simulink model "bike_model_old"  (R2018b)
settings: Solver=VariableStepAuto  StartTime=0.0  StopTime=sim_time  FixedStep=Ts_IMU  MaxStep=Ts  RelTol=1e-3
values from neighbouring files (symbols this model uses):
  a_compFilter = b_compFilter - 0.77    (= 0.325)    [configuration.m]    (also in configuration_pidTuning.m)
  A_kalman = [1 0 Ts 0; 0 1 0 Ts; 0 0 1 0; 0 0 0 1]    [configuration.m]    (also in configuration_pidTuning.m)
  b_compFilter = 1.095    [configuration.m]    (also in configuration_pidTuning.m)
  B_kalman = [0 0 0 0; 0 0 0 0; 0 0 0 0; 0 0 0 0]    [configuration.m]    (also in configuration_pidTuning.m)
  b_real = 1.095    [configuration.m]    (also in configuration_pidTuning.m)
  C_kalman = [1 0 0 0; 0 1 0 0; 0 0 1 0; 0 0 0 1]    [configuration.m]    (also in configuration_pidTuning.m)
  complementary = 0.985    [configuration.m]    (also in configuration_pidTuning.m)
  D_kalman = [0 0 0 0; 0 0 0 0; 0 0 0 0; 0 0 0 0]    [configuration.m]    (also in configuration_pidTuning.m)
  Dead_Band = [0.055, -0.055, 0.005]    [configuration.m]    (also in configuration_pidTuning.m)
  delay = 0.045    [configuration.m]    (also in configuration_pidTuning.m)
  direct_control = 1    [configuration.m]    (also in configuration_pidTuning.m)
  filter_model = 1    [configuration.m]    (also in configuration_pidTuning.m)
  forward_motor_dynamics = 0    [configuration.m]    (also in configuration_pidTuning.m)
  forward_speed_offset = 0    [configuration.m]
  g = 9.81    [configuration.m]    (also in configuration_pidTuning.m)
  I_direct = 0.000227125326188444    (= 0.000227125326188)    [configuration.m]    (also in configuration_pidTuning.m)
  I_lat = 0.000115580509653549    (= 0.000115580509654)    [configuration.m]    (also in configuration_pidTuning.m)
  I_steer = 0.4510120195392    (= 0.451012019539)    [configuration.m]    (also in configuration_pidTuning.m)
  IMU_height_model = 0.45    [configuration.m]    (also in configuration_pidTuning.m)
  IMU_height_real = 0.45    [configuration.m]    (also in configuration_pidTuning.m)
  initial_states = [deg2rad(-2) deg2rad(0) deg2rad(0)]    [configuration.m]    (also in configuration_pidTuning.m)
  input_velocity = 4    [configuration.m]    (also in configuration_pidTuning.m = 3)
  K_dir = [0.2 0 0]    [configuration.m]
  K_pos = [0.02 0 0]    [configuration.m]
  lambda_compFilter = deg2rad(70)    [configuration.m]    (also in configuration_pidTuning.m)
  lambda_real = deg2rad(70)    [configuration.m]    (also in configuration_pidTuning.m)
  lat_control = 0    [configuration.m]    (also in configuration_pidTuning.m = 1)
  look_ahead = 0    [configuration.m]    (also in configuration_pidTuning.m)
  lqr_gains = zeros(length(velocity_lqr),1+size(A_bike,1))    [lqr_design.m]
  max_handlebar = 40*(pi/180)    (= 0.698131700798)    [configuration.m]    (also in configuration_pidTuning.m)
  max_roll = pi/2    (= 1.57079632679)    [configuration.m]    (also in configuration_pidTuning.m)
  max_steering_motor_acc = inf    [configuration.m]    (also in configuration_pidTuning.m)
  max_steering_motor_speed = 0.9    [configuration.m]    (also in configuration_pidTuning.m = 7.5)
  min_handlebar = -max_handlebar    (= -0.698131700798)    [configuration.m]    (also in configuration_pidTuning.m)
  min_roll = - max_roll    (= -1.57079632679)    [configuration.m]    (also in configuration_pidTuning.m)
  min_steering_motor_acc = -inf    [configuration.m]    (also in configuration_pidTuning.m)
  min_steering_motor_speed = -0.9    [configuration.m]    (also in configuration_pidTuning.m = -7.5)
  noise = 0    [configuration.m]    (also in configuration_pidTuning.m)
  noise_acc = 2.4869e-05    [configuration.m]    (also in configuration_pidTuning.m)
  noise_encoder = 1e-7    (= 1e-07)    [configuration.m]    (also in configuration_pidTuning.m)
  noise_gyro = 0.005    [configuration.m]    (also in configuration_pidTuning.m = 0.0022)
  noise_hall = 0.0031    [configuration.m]    (also in configuration_pidTuning.m)
  noise_pos_meas = 0    [configuration.m]    (also in configuration_pidTuning.m = 0.51)
  offset_acc = 0.0*g    (= 0)    [configuration.m]
  offset_encoder = deg2rad(1)    [configuration.m]
  offset_gyro = deg2rad(0)    [configuration.m]
  offset_hall = 0.0    (= 0)    [configuration.m]
  offset_pos_x = 0    [configuration.m]
  offset_pos_y = 0    [configuration.m]
  P_direct = 0.0712859744206787    (= 0.0712859744207)    [configuration.m]    (also in configuration_pidTuning.m)
  P_lat = 0.0465435246389258    (= 0.0465435246389)    [configuration.m]    (also in configuration_pidTuning.m)
  P_steer = 0.219020351848633    (= 0.219020351849)    [configuration.m]    (also in configuration_pidTuning.m)
  parameters_compFilter = [g h_compFilter b_compFilter a_compFilter lambda_compFilter c_compFilter]    [configuration.m]    (also in configuration_pidTuning.m)
  parameters_f_b_real = [m_frame_real m_box_real h_frame_real h_box_real a_frame_real a_box_real c_frame_real c_box_real b_frame_real b_box_real l_frame_real l_box_real]    [configuration.m]    (also in configuration_pidTuning.m)
  parameters_real = [g h_real b_real a_real lambda_real c_real]    [configuration.m]    (also in configuration_pidTuning.m)
  path_tracking = 0    [configuration.m]    (also in configuration_pidTuning.m = 1)
  plant_model = 2    [configuration.m]    (also in configuration_pidTuning.m = 1)
  R_kalman = [noise_pos_meas 0 0 0; 0 noise_pos_meas 0 0; 0 0 noise_hall 0; 0 0 0 noise_hall]    [configuration.m]    (also in configuration_pidTuning.m)
  roll_rate_coef = 0.9    [configuration.m]    (also in configuration_pidTuning.m)
  sensor_offset = 0    [configuration.m]
  steer_control = 0    [configuration.m]    (also in configuration_pidTuning.m = 1)
  steering_angle_correction = deg2rad(0)    [configuration.m]
  steering_motor_limitations = 0    [configuration.m]    (also in configuration_pidTuning.m = 1)
  sys_con = ss(A_lqr,B_lqr,C_lqr,D_lqr)    [lqr_design.m]
  sys_dis = c2d(sys_con,Ts)    [lqr_design.m]
  time_offset_acc = 7    [configuration.m]
  time_offset_encoder = 10    [configuration.m]
  time_offset_gyro = 7    [configuration.m]
  time_offset_hall = 7    [configuration.m]
  time_offset_pos_x = 7    [configuration.m]
  time_offset_pos_y = 7    [configuration.m]
  Ts = 0.01    [configuration.m]    (also in configuration_pidTuning.m = 0.04)
  Ts_IMU = 0.01    [configuration.m]    (also in configuration_pidTuning.m = 0.04)
  uneven_mass = 0    [configuration.m]
  velocity_lqr = [input_velocity - 0.1 , input_velocity , input_velocity + 0.1]    [lqr_design.m]
undefined symbols (not defined in the file or in its folder): A, B, cumulative_dist_along_path, curvature, DiscIntNeverNeededParam, Discrete, initial_x, initial_y, path_x, path_y, Time
libraries: simulink x23, simulink_extras x4, dspsigops x2, ctrlSharedLib x1
(part 1 of 3)
settings Model: Creator=Boaz Ash  LastModifiedBy=maximef
settings DebuggingCC: UnconnectedInputMsg=none  UnconnectedOutputMsg=none  UnconnectedLineMsg=none  LibraryContextMissingDiagnostic=none
settings SFSimCC: SimUseLocalCustomCode=off
settings RTWCC: RTWUseLocalCustomCode=off

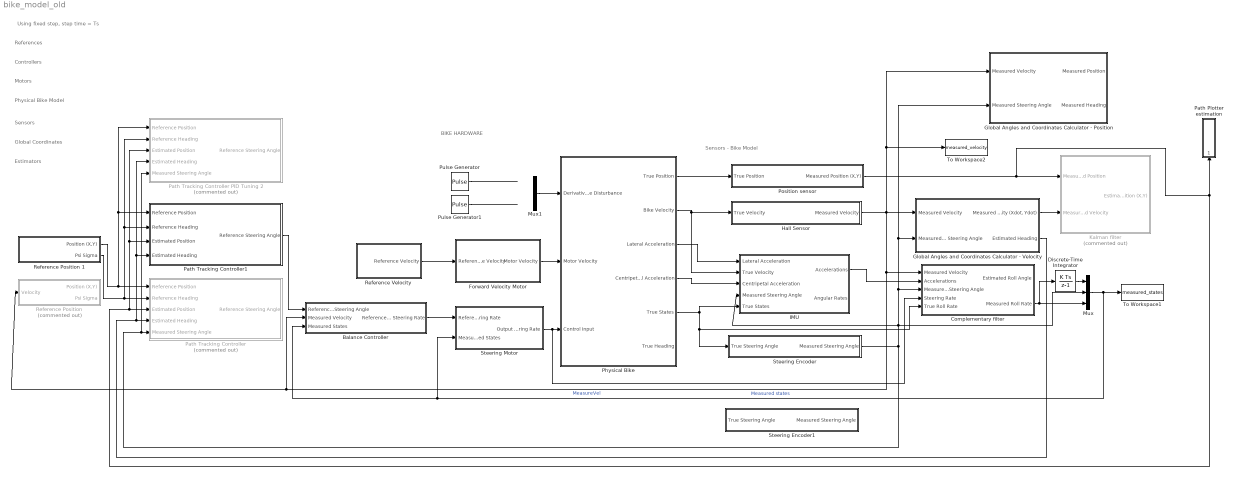
== system bike_model_old ==
  note: Using fixed step, step time = Ts
  note: BIKE HARDWARE
  note: References
  note: Physical Bike
      | Model
  note: Sensors - Bike Model
  note: Motors
  note: Sensors
  note: Global Coordinates
  note: Controllers
  note: Estimators
  Balance Controller : Subsystem  TreatAsAtomicUnit=on  SystemSampleTime=Ts
  Complementary filter : Subsystem  SystemSampleTime=Ts_IMU
  Discrete-Time Integrator : DiscreteIntegrator  SampleTime=Ts  ICPrevOutput=DiscIntNeverNeededParam  ICPrevScaledInput=DiscIntNeverNeededParam
  Forward Velocity Motor : Subsystem
  Global Angles and Coordinates Calculator - Position : Subsystem  SystemSampleTime=Ts
  Global Angles and Coordinates Calculator - Velocity : Subsystem  SystemSampleTime=Ts
  Hall Sensor : Subsystem  TreatAsAtomicUnit=on  SystemSampleTime=Ts
  IMU : Subsystem  TreatAsAtomicUnit=on
  "Kalman filter " : Subsystem  Commented=on  SystemSampleTime=Ts
  Mux : Mux  Inputs=3
  Mux1 : Mux  Inputs=3
  Path Plotter estimation : Subsystem  SystemSampleTime=Ts
  Path Tracking Controller : Subsystem  Commented=on
  Path Tracking Controller PID Tuning 2 : Subsystem  Commented=on
  Path Tracking Controller1 : Subsystem
  Physical Bike : Subsystem
  Position sensor : Subsystem  TreatAsAtomicUnit=on  SystemSampleTime=Ts
  Pulse Generator : DiscretePulseGenerator  PulseType=Time based  Amplitude=pi/36  Period=100  PhaseDelay=1
  Pulse Generator1 : DiscretePulseGenerator  PulseType=Time based  Amplitude=-deg2rad(30)  Period=10  PulseWidth=10  PhaseDelay=1
  "Reference Position " : Subsystem  Commented=on
  Reference Position 1 : Subsystem
  "Reference Velocity " : Subsystem
  Steering Encoder : Subsystem  TreatAsAtomicUnit=on  SystemSampleTime=Ts
  Steering Encoder1 : Subsystem  TreatAsAtomicUnit=on  SystemSampleTime=Ts
  Steering Motor : Subsystem
  To Workspace1 : ToWorkspace  VariableName=measured_states  SaveFormat=Timeseries  SampleTime=-1
  To Workspace2 : ToWorkspace  VariableName=measured_velocity  SaveFormat=Timeseries  SampleTime=-1
  wires:
  Mux1/1 -> Physical Bike/1(Derivative Disturbance)
  "Reference Velocity "/1(Reference Velocity) -> Forward Velocity Motor/1(Reference Velocity)
  Forward Velocity Motor/1(Motor Velocity) -> Physical Bike/2(Motor Velocity)
  Pulse Generator/1 -> ?
  Pulse Generator1/1 -> ?
  Position sensor/1("Measured Position (X,Y) ") -> Path Tracking Controller1/3(Estimated Position), Path Tracking Controller PID Tuning 2/3(Estimated Position), Path Tracking Controller/3(Estimated Position), Path Plotter estimation/1(Position), "Kalman filter "/1("Measured Position ")
  Global Angles and Coordinates Calculator - Velocity/2(Estimated Heading) -> Path Tracking Controller PID Tuning 2/4(Estimated Heading), Path Tracking Controller1/4(Estimated Heading), Path Tracking Controller/4(Estimated Heading)
  Path Tracking Controller1/1(Reference Steering Angle) -> Balance Controller/1(Reference Steering Angle)
  Balance Controller/1(Reference Steering Rate) -> Steering Motor/1(Reference Steering Rate)
  Physical Bike/3(Lateral Acceleration) -> IMU/1(Lateral Acceleration)
  Physical Bike/4(Centripetal Acceleration) -> IMU/3(Centripetal Acceleration)
  Mux/1 -> To Workspace1/1, Steering Motor/2(Measured States), Balance Controller/3(Measured States)  "Measured states"
  Steering Encoder/1(Measured Steering Angle) -> Global Angles and Coordinates Calculator - Position/2(Measured Steering Angle), Global Angles and Coordinates Calculator - Velocity/2("Measured Steering Angle "), Complementary filter/3(Measured Steering Angle), Mux/2, IMU/4(Measured Steering Angle), Path Tracking Controller PID Tuning 2/5(Measured Steering Angle), Path Tracking Controller/5(Measured Steering Angle)
  IMU/1(Accelerations) -> Complementary filter/2(Accelerations)
  Global Angles and Coordinates Calculator - Velocity/1("Measured Velocity (Xdot, Ydot)") -> "Kalman filter "/2(Measured Velocity)
  Hall Sensor/1(Measured Velocity) -> Global Angles and Coordinates Calculator - Position/1(Measured Velocity), To Workspace2/1, Complementary filter/1(Measured Velocity), Balance Controller/2(Measured Velocity), "Reference Position "/1(Velocity), Global Angles and Coordinates Calculator - Velocity/1(Measured Velocity)  "MeasureVel"
  Reference Position 1/2(Psi Sigma) -> Path Tracking Controller1/2(Reference Heading), Path Tracking Controller PID Tuning 2/2(Reference Heading), Path Tracking Controller/2(Reference Heading)
  Reference Position 1/1(Position (X,Y)) -> Path Tracking Controller PID Tuning 2/1(Reference Position), Path Tracking Controller1/1(Reference Position), Path Tracking Controller/1(Reference Position)
  Physical Bike/2(Bike Velocity) -> IMU/2(True Velocity), Hall Sensor/1(True Velocity)
  Physical Bike/1(True Position) -> Position sensor/1(True Position)
  Steering Motor/1(Output Steering Rate) -> Complementary filter/4(Steering Rate), Physical Bike/3(Control Input)
  Physical Bike/5(True States) -> Complementary filter/5(True Roll Rate), Steering Encoder/1(True Steering Angle), IMU/5(True States)
  Complementary filter/2(Measured Roll Rate) -> Mux/3, Discrete-Time Integrator/1
  Discrete-Time Integrator/1 -> Mux/1

== system bike_model_old/Balance Controller ==
  Reference Steering Angle : Inport
  Measured Velocity : Inport  Port=2
  Measured States : Inport  Port=3
  LQR Controller : Subsystem  TreatAsAtomicUnit=on  SystemSampleTime=Ts
  Reference States : Subsystem  SystemSampleTime=Ts
  Sum : Sum  Inputs=|+-
  To Workspace : ToWorkspace  VariableName=states_measured  SaveFormat=Timeseries  SampleTime=-1
  Reference Steering Rate : Outport
  wires:
  Reference States/1(Reference States) -> Sum/1
  Sum/1 -> LQR Controller/2(State Error)
  LQR Controller/1(Calculated Input) -> Reference Steering Rate/1
  Measured Velocity/1 -> Reference States/1(Velocity), LQR Controller/1(Velocity)
  Measured States/1 -> To Workspace/1, Sum/2
  Reference Steering Angle/1 -> Reference States/2(Delta Ref)

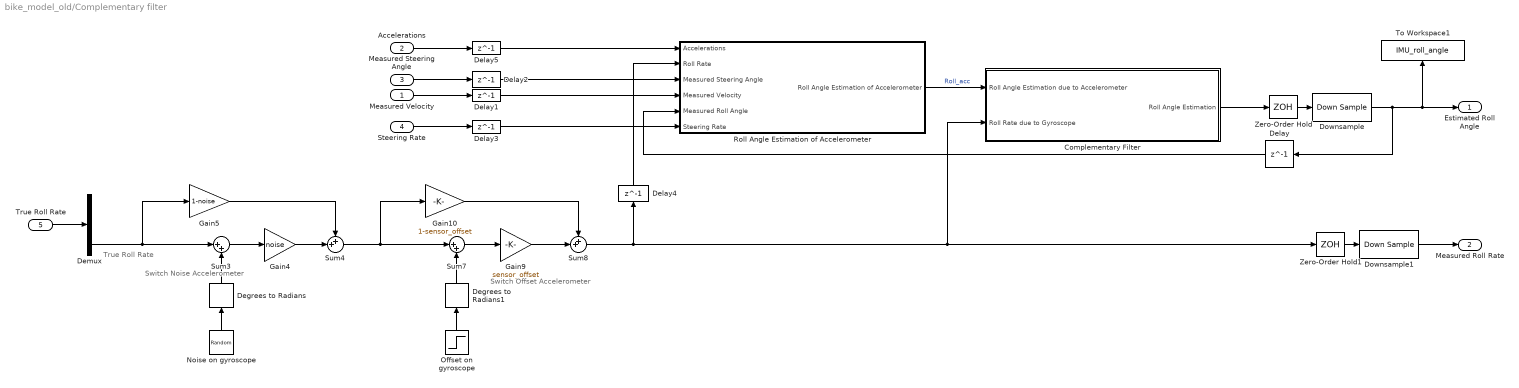
== system bike_model_old/Complementary filter ==
  note: Switch Noise
      | Accelerometer
  note: True Roll
      | Rate
  note: Switch Offset
      | Accelerometer
  Measured Velocity : Inport
  Accelerations : Inport  Port=2
  Measured Steering Angle : Inport  Port=3
  Steering Rate : Inport  Port=4
  True Roll Rate : Inport  Port=5
  Complementary Filter : Subsystem  TreatAsAtomicUnit=on  SystemSampleTime=Ts_IMU
  Degrees to Radians : simulink_extras/Transformations/Degrees to Radians
  Degrees to Radians1 : simulink_extras/Transformations/Degrees to Radians
  Delay{,1..2,4..5} (5 alike) : Delay  DelayLength=1
  Delay3 : Delay  DelayLength=1  SampleTime=Ts_IMU
  Demux : Demux  Outputs=3
  Downsample : DownSample  N=Ts/Ts_IMU  RateOptions=Allow multirate processing
  Downsample1 : DownSample  N=Ts/Ts_IMU  RateOptions=Allow multirate processing
  Gain10 : Gain  Gain=1-sensor_offset
  Gain4 : Gain  Gain=noise
  Gain5 : Gain  Gain=1-noise
  Gain9 : Gain  Gain=sensor_offset
  Noise on gyroscope : RandomNumber  Variance=noise_gyro  SampleTime=Ts
  Offset on gyroscope : Step  Time=time_offset_gyro  After=offset_gyro  SampleTime=Ts
  Roll Angle Estimation of Accelerometer : Subsystem
  Sum3 : Sum  Inputs=|++
  Sum4 : Sum  Inputs=++|
  Sum7 : Sum  Inputs=|++
  Sum8 : Sum  Inputs=++|
  To Workspace1 : ToWorkspace  VariableName=IMU_roll_angle  SaveFormat=Structure  SampleTime=-1
  Zero-Order Hold : ZeroOrderHold  SampleTime=Ts_IMU
  Zero-Order Hold1 : ZeroOrderHold  SampleTime=Ts_IMU
  Estimated Roll Angle : Outport
  Measured Roll Rate : Outport  Port=2
  wires:
  Roll Angle Estimation of Accelerometer/1(Roll Angle Estimation of Accelerometer) -> Complementary Filter/1(Roll Angle Estimation due to Accelerometer)  "Roll_acc"
  Sum8/1 -> Zero-Order Hold1/1, Complementary Filter/2(Roll Rate due to Gyroscope), Delay4/1
  Zero-Order Hold/1 -> Downsample/1
  Zero-Order Hold1/1 -> Downsample1/1
  Accelerations/1 -> Delay5/1
  Measured Steering Angle/1 -> Delay2/1
  Measured Velocity/1 -> Delay1/1
  Delay/1 -> Roll Angle Estimation of Accelerometer/5(Measured Roll Angle)
  Delay1/1 -> Roll Angle Estimation of Accelerometer/4(Measured Velocity)
  Delay2/1 -> Roll Angle Estimation of Accelerometer/3(Measured Steering Angle)
  Steering Rate/1 -> Delay3/1
  Delay3/1 -> Roll Angle Estimation of Accelerometer/6(Steering Rate)
  Delay4/1 -> Roll Angle Estimation of Accelerometer/2(Roll Rate)
  Delay5/1 -> Roll Angle Estimation of Accelerometer/1(Accelerations)
  Complementary Filter/1(Roll Angle Estimation) -> Zero-Order Hold/1
  Downsample1/1 -> Measured Roll Rate/1
  Downsample/1 -> Estimated Roll Angle/1, To Workspace1/1, Delay/1
  Demux/3 -> Sum3/1, Gain5/1
  Sum3/1 -> Gain4/1
  Noise on gyroscope/1 -> Degrees to Radians/1
  Gain4/1 -> Sum4/2
  Gain5/1 -> Sum4/1
  Degrees to Radians/1 -> Sum3/2
  True Roll Rate/1 -> Demux/1
  Gain9/1 -> Sum8/2
  Sum7/1 -> Gain9/1
  Sum4/1 -> Gain10/1, Sum7/1
  Degrees to Radians1/1 -> Sum7/2
  Offset on gyroscope/1 -> Degrees to Radians1/1
  Gain10/1 -> Sum8/1

== system bike_model_old/Forward Velocity Motor ==
  note: Add limit for acceleration/deceleration
      | Add min speed of 1.69 m/s (3600 rpm motor speed) limitation
      | Add min speed of 8.20 m/s (18000 rpm motor speed) limitation
      | Add deadband and delay
  Reference Velocity : Inport
  Band-Limited White Noise : simulink/Sources/Band-Limited White Noise  Cov=[0.001]  Ts=Ts  seed=[23341]
  Constant : Constant  Value=forward_motor_dynamics
  Rate Limiter : RateLimiter  RisingSlewLimit=inf  FallingSlewLimit=-inf  SampleTimeMode=inherited
  Saturation : Saturate  UpperLimit=inf  LowerLimit=0
  Sum : Sum  Inputs=|++
  Switch : Switch  Criteria=u2 > Threshold
  Transfer Fcn : TransferFcn  Numerator=[-0.2156 0.556]  Denominator=[1 1.675 0.5558]
  Motor Velocity : Outport
  wires:
  Reference Velocity/1 -> Transfer Fcn/1, Switch/3
  Transfer Fcn/1 -> Rate Limiter/1
  Switch/1 -> Sum/1
  Constant/1 -> Switch/2
  Saturation/1 -> Switch/1
  Rate Limiter/1 -> Saturation/1
  Sum/1 -> Motor Velocity/1

== system bike_model_old/Global Angles and Coordinates Calculator - Position ==
  note: True Steering
      | Angle
  Measured Velocity : Inport
  Measured Steering Angle : Inport  Port=2
  Gain1 : Gain  Gain=sin(lambda_compFilter)
  Measured Bike Angles to Global Angles : Subsystem
  Measured Global Angles to Global Coordinates : Subsystem
  Sum : Sum  Inputs=++|
  Measured Position : Outport
  Measured Heading : Outport  Port=2
  wires:
  Measured Bike Angles to Global Angles/1(Psi) -> Sum/2, Measured Global Angles to Global Coordinates/2(Psi)
  Gain1/1 -> Measured Bike Angles to Global Angles/2(Measured Steering Angle)
  Sum/1 -> Measured Heading/1
  Measured Bike Angles to Global Angles/2(Beta) -> Sum/1, Measured Global Angles to Global Coordinates/3(Beta)
  Measured Global Angles to Global Coordinates/1("Position (X, Y)") -> Measured Position/1
  Measured Velocity/1 -> Measured Global Angles to Global Coordinates/1(Velocity), Measured Bike Angles to Global Angles/1(Velocity)
  Measured Steering Angle/1 -> Gain1/1

== system bike_model_old/Global Angles and Coordinates Calculator - Velocity ==
  Measured Velocity : Inport
  "Measured Steering Angle " : Inport  Port=2
  Gain1 : Gain  Gain=sin(lambda_compFilter)
  Measured Bike Angles to Global Angles : Subsystem
  Measured Global Angles to Global Coordinates : Subsystem
  Sum : Sum  Inputs=++|
  "Measured Velocity (Xdot, Ydot)" : Outport
  Estimated Heading : Outport  Port=2
  wires:
  "Measured Steering Angle "/1 -> Gain1/1
  Measured Bike Angles to Global Angles/1(Psi) -> Sum/2, Measured Global Angles to Global Coordinates/2(Psi)
  Gain1/1 -> Measured Bike Angles to Global Angles/2(Measured Steering Angle)
  Sum/1 -> Estimated Heading/1
  Measured Bike Angles to Global Angles/2(Beta) -> Measured Global Angles to Global Coordinates/3(Beta), Sum/1
  Measured Velocity/1 -> Measured Bike Angles to Global Angles/1(Velocity), Measured Global Angles to Global Coordinates/1(Velocity)
  Measured Global Angles to Global Coordinates/1("Velocity (Xdot, Ydot)") -> "Measured Velocity (Xdot, Ydot)"/1

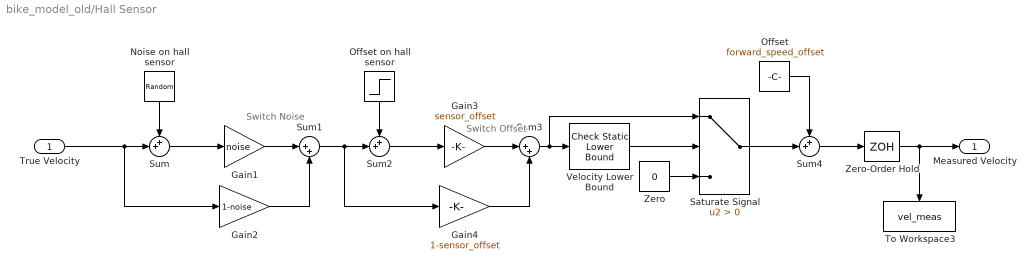
== system bike_model_old/Hall Sensor ==
  note: Switch Noise
  note: Switch Offset
  True Velocity : Inport
  Gain1 : Gain  Gain=noise
  Gain2 : Gain  Gain=1-noise
  Gain3 : Gain  Gain=sensor_offset
  Gain4 : Gain  Gain=1-sensor_offset
  Noise on hall sensor : RandomNumber  Variance=noise_hall  SampleTime=Ts
  Offset : Constant  Value=forward_speed_offset
  Offset on hall sensor : Step  Time=time_offset_hall  After=offset_hall  SampleTime=Ts
  Saturate Signal : Switch  Criteria=u2 > Threshold
  Sum : Sum  Inputs=++|
  Sum1 : Sum  Inputs=|++
  Sum2 : Sum  Inputs=++|
  Sum3 : Sum  Inputs=|++
  Sum4 : Sum  Inputs=++|
  To Workspace3 : ToWorkspace  VariableName=vel_meas  SaveFormat=Timeseries  SampleTime=-1
  Velocity Lower Bound : simulink/Model Verification/Check Static  Lower Bound  Description=0.6 <= u  min=0.6  min_included=on  enabled=on  stopWhenAssertionFail=off  export=on  icon=graphic
      settings: SourceProductName=Simulink
  Zero : Constant  Value=0
  Zero-Order Hold : ZeroOrderHold  SampleTime=Ts
  Measured Velocity : Outport
  wires:
  Sum3/1 -> Saturate Signal/1, Velocity Lower Bound/1
  Noise on hall sensor/1 -> Sum/1
  Zero/1 -> Saturate Signal/3
  Velocity Lower Bound/1 -> Saturate Signal/2
  True Velocity/1 -> Gain2/1, Sum/2
  Gain1/1 -> Sum1/1
  Gain2/1 -> Sum1/2
  Sum/1 -> Gain1/1
  Sum1/1 -> Gain4/1, Sum2/2
  Sum2/1 -> Gain3/1
  Gain4/1 -> Sum3/2
  Gain3/1 -> Sum3/1
  Offset on hall sensor/1 -> Sum2/1
  Sum4/1 -> Zero-Order Hold/1
  Offset/1 -> Sum4/1
  Saturate Signal/1 -> Sum4/2
  Zero-Order Hold/1 -> To Workspace3/1, Measured Velocity/1

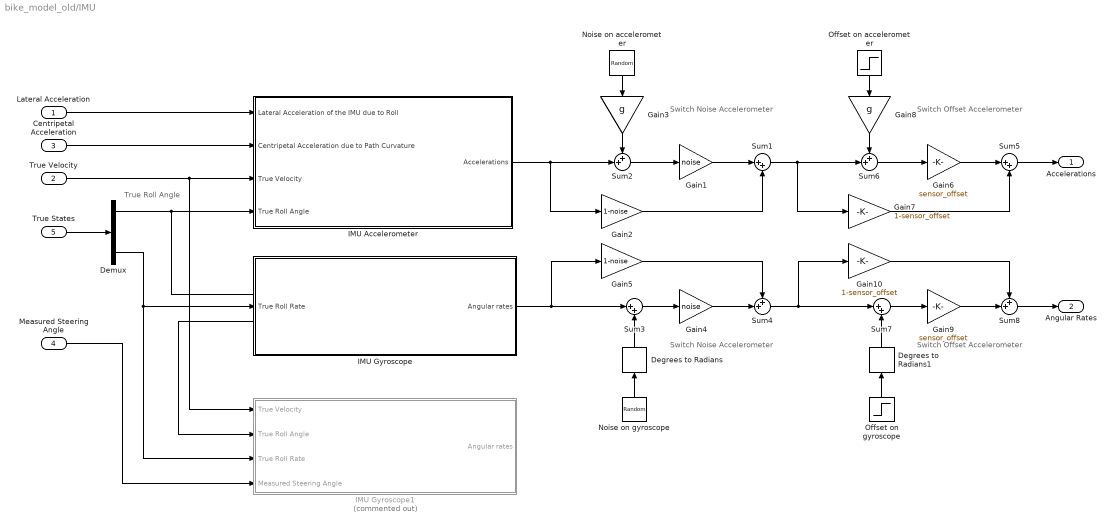
== system bike_model_old/IMU ==
  note: True Roll
      | Angle
  note: Switch Noise
      | Accelerometer
  note: Switch Noise
      | Accelerometer
  note: Switch Offset
      | Accelerometer
  note: Switch Offset
      | Accelerometer
  Lateral Acceleration : Inport
  True Velocity : Inport  Port=2
  Centripetal Acceleration : Inport  Port=3
  Measured Steering Angle : Inport  Port=4
  True States : Inport  Port=5
  Degrees to Radians : simulink_extras/Transformations/Degrees to Radians
  Degrees to Radians1 : simulink_extras/Transformations/Degrees to Radians
  Demux : Demux  Outputs=3
  Gain1 : Gain  Gain=noise
  Gain10 : Gain  Gain=1-sensor_offset
  Gain2 : Gain  Gain=1-noise
  Gain3 : Gain  Gain=g
  Gain4 : Gain  Gain=noise
  Gain5 : Gain  Gain=1-noise
  Gain6 : Gain  Gain=sensor_offset
  Gain7 : Gain  Gain=1-sensor_offset
  Gain8 : Gain  Gain=g
  Gain9 : Gain  Gain=sensor_offset
  IMU Accelerometer : Subsystem
  IMU Gyroscope : Subsystem
  IMU Gyroscope1 : Subsystem  Commented=on
  Noise on accelerometer : RandomNumber  Variance=noise_acc  SampleTime=Ts
  Noise on gyroscope : RandomNumber  Variance=noise_gyro  SampleTime=Ts
  Offset on accelerometer : Step  Time=time_offset_acc  After=offset_acc  SampleTime=Ts
  Offset on gyroscope : Step  Time=time_offset_gyro  After=offset_gyro  SampleTime=Ts
  Sum{1,3,5,7} (4 alike) : Sum  Inputs=|++
  Sum{2,4,6,8} (4 alike) : Sum  Inputs=++|
  Accelerations : Outport
  Angular Rates : Outport  Port=2
  wires:
  Measured Steering Angle/1 -> IMU Gyroscope1/4(Measured Steering Angle)
  True Velocity/1 -> IMU Gyroscope1/1(True Velocity), IMU Accelerometer/3(True Velocity)
  Lateral Acceleration/1 -> IMU Accelerometer/1(Lateral Acceleration of the IMU due to Roll)
  Centripetal Acceleration/1 -> IMU Accelerometer/2(Centripetal Acceleration due to Path Curvature)
  True States/1 -> Demux/1
  Demux/1 -> IMU Gyroscope1/2(True Roll Angle), IMU Accelerometer/4(True Roll Angle)
  Gain2/1 -> Sum1/2
  IMU Accelerometer/1(Accelerations) -> Sum2/2, Gain2/1
  Noise on accelerometer/1 -> Gain3/1
  Gain3/1 -> Sum2/1
  Noise on gyroscope/1 -> Degrees to Radians/1
  IMU Gyroscope/1(Angular rates) -> Sum3/1, Gain5/1
  Degrees to Radians/1 -> Sum3/2
  Gain5/1 -> Sum4/1
  Sum3/1 -> Gain4/1
  Gain4/1 -> Sum4/2
  Sum2/1 -> Gain1/1
  Gain1/1 -> Sum1/1
  Gain10/1 -> Sum8/1
  Sum4/1 -> Sum7/1, Gain10/1
  Offset on gyroscope/1 -> Degrees to Radians1/1
  Degrees to Radians1/1 -> Sum7/2
  Sum7/1 -> Gain9/1
  Sum6/1 -> Gain6/1
  Gain8/1 -> Sum6/1
  Sum1/1 -> Sum6/2, Gain7/1
  Gain6/1 -> Sum5/1
  Gain9/1 -> Sum8/2
  Offset on accelerometer/1 -> Gain8/1
  Gain7/1 -> Sum5/2
  Sum5/1 -> Accelerations/1
  Sum8/1 -> Angular Rates/1
  Demux/3 -> IMU Gyroscope1/3(True Roll Rate), IMU Gyroscope/1(True Roll Rate)

== system bike_model_old/Kalman filter  ==
  note: y_k
  note: Measurements
  "Measured Position " : Inport
  Measured Velocity : Inport  Port=2
  Demux : Demux  Outputs=2
  "Kalman Filter " : ctrlSharedLib/Kalman Filter  TimeDomain=Discrete-Time  UseCurrentEstimator=on  ModelSource=Individual A, B, C, D matrices  ModelSourceVariable=ss(0.95,1,1,0,1)  A=A_kalman  B=B_kalman  C=C_kalman  D=D_kalman  NumberOfStates=1  NumberOfInputs=1  NumberOfOutputs=1  InitialEstimateSource=Dialog  X0=0  P0=10  UseK=off  UseGH=off  NumberOfProcessNoiseInputs=1  G=1  TimeInvariantG=on  H=0  TimeInvariantH=on  Q=Q_kalman  TimeInvariantQ=on  R=R_kalman  TimeInvariantR=on  N=0  TimeInvariantN=on  AddInputPort=on  AddEnablePort=off  OutputEstimatedY=off  OutputP=off  Ts=Ts
      settings: SourceProductBaseCode=CT
  Mux : Mux  Inputs=2
  Zero-Order Hold : ZeroOrderHold  SampleTime=-1
  Estimated Position (X,Y) : Outport
  wires:
  Measured Velocity/1 -> Mux/2
  Mux/1 -> Zero-Order Hold/1
  "Measured Position "/1 -> Mux/1
  "Kalman Filter "/1 -> Demux/1
  Demux/1 -> Estimated Position (X,Y)/1
  Zero-Order Hold/1 -> "Kalman Filter "/2

== system bike_model_old/Path Plotter estimation ==
  Position : Inport
  Demux : Demux  Outputs=2
  To Workspace : ToWorkspace  VariableName=X_BIKE_estim  SaveFormat=Timeseries  SampleTime=Ts
  To Workspace1 : ToWorkspace  VariableName=Y_BIKE_estim  SaveFormat=Timeseries  SampleTime=Ts
  XY Graph : simulink/Sinks/XY Graph  Commented=on  xmin=min(path_x)-5  xmax=max(path_x)+5  ymin=min(path_y)-5  ymax=max(path_y)+5  st=-1
  wires:
  Demux/1 -> XY Graph/1, To Workspace/1  "X"
  Demux/2 -> XY Graph/2, To Workspace1/1  "Y"
  Position/1 -> Demux/1

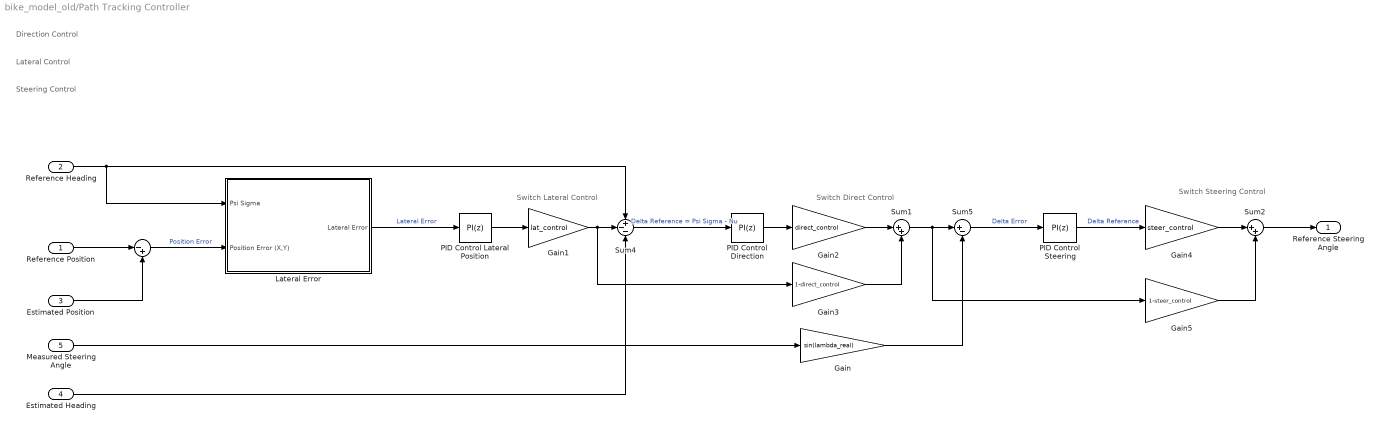
== system bike_model_old/Path Tracking Controller ==
  note: Switch Steering Control
  note: Direction Control
  note: Lateral Control
  note: Steering Control
  note: Switch Direct Control
  note: Switch Lateral Control
  Reference Position : Inport
  Reference Heading : Inport  Port=2
  Estimated Position : Inport  Port=3
  Estimated Heading : Inport  Port=4
  Measured Steering Angle : Inport  Port=5
  " " : Sum  Inputs=|-+
  Gain : Gain  Gain=sin(lambda_real)
  Gain1 : Gain  Gain=lat_control
  Gain2 : Gain  Gain=direct_control
  Gain3 : Gain  Gain=1-direct_control
  Gain4 : Gain  Gain=steer_control
  Gain5 : Gain  Gain=1-steer_control
  Lateral Error : Subsystem  SystemSampleTime=Ts
  PID Control Lateral Position : simulink/Continuous/PID Controller  Controller=PI  Form=Parallel  TimeDomain=Discrete-time  SampleTime=Ts  IntegratorMethod=Forward Euler  FilterMethod=Forward Euler  ControllerParametersSource=internal  P=P_lat  I=I_lat  D=0  UseFilter=on  N=100  TunerSelectOption=Transfer Function Based (PID Tuner App)  InitialConditionSource=internal  InitialConditionForIntegrator=0  InitialConditionForFilter=0  DifferentiatorICPrevScaledInput=0  ExternalReset=none  TrackingMode=off  Kt=1  LimitOutput=off  UpperSaturationLimit=inf  LowerSaturationLimit=-inf  LinearizeAsGain=on  AntiWindupMode=none  Kb=1  POutMin=[]  POutMax=[]  IOutMin=[]  IOutMax=[]  DOutMin=[]  DOutMax=[]  NOutMin=[]  NOutMax=[]  SumOutMin=[]  SumOutMax=[]  SaturationOutMin=[]  SaturationOutMax=[]  PParamMin=[]  PParamMax=[]  IParamMin=[]  IParamMax=[]  DParamMin=[]  DParamMax=[]  NParamMin=[]  NParamMax=[]  KbParamMin=[]  KbParamMax=[]  KtParamMin=[]  KtParamMax=[]  KbOutMin=[]  KbOutMax=[]  KtOutMin=[]  KtOutMax=[]  IntegratorOutMin=[]  IntegratorOutMax=[]  FilterOutMin=[]  FilterOutMax=[]  SumI1OutMin=[]  SumI1OutMax=[]  SumI2OutMin=[]  SumI2OutMax=[]  SumI3OutMin=[]  SumI3OutMax=[]  SumI4OutMin=[]  SumI4OutMax=[]  SumDOutMin=[]  SumDOutMax=[]  DifferentiatorOutMin=[]  DifferentiatorOutMax=[]  FilterDiffOutCoefMin=[]  FilterDiffOutCoefMax=[]  ReciprocalOutMin=[]  ReciprocalOutMax=[]  SumDenOutMin=[]  SumDenOutMax=[]  SumNumOutMin=[]  SumNumOutMax=[]  DivideOutMin=[]  DivideOutMax=[]  IntegratorContinuousStateAttributes=''  IntegratorStateMustResolveToSignalObject=off  IntegratorRTWStateStorageClass=Auto  FilterContinuousStateAttributes=''  FilterStateMustResolveToSignalObject=off  FilterRTWStateStorageClass=Auto  ParallelPVariant=InternalParameters  IdealPVariant=Disabled  IVariant=InternalParameters  DVariant=Disabled  IntegratorVariant=Discrete  SatVariant=Disabled  AWVariant=Passthrough  PCopyVariant=Disabled  TRVariant=Disabled  FdbkBlocksVariant=Forward  IdealPFdbkVariant=Disabled  SatFdbkVariant=Disabled  DerivativeFilterVariant=Disabled  NVariant=Disabled  NCopyVariant=Disabled_SignalSpec  FilterICVariant=Disabled  IntegratorICVariant=InternalICs  ExternalResetVariant=Disabled  TRSumVariant=Passthrough  SumFdbkVariant=Disabled  SumVariant=Sum_PI
  PID Control Direction : simulink/Continuous/PID Controller  Controller=PI  Form=Parallel  TimeDomain=Discrete-time  SampleTime=Ts  IntegratorMethod=Forward Euler  FilterMethod=Forward Euler  ControllerParametersSource=internal  P=P_direct  I=I_direct  D=0  UseFilter=on  N=100  TunerSelectOption=Transfer Function Based (PID Tuner App)  InitialConditionSource=internal  InitialConditionForIntegrator=0  InitialConditionForFilter=0  DifferentiatorICPrevScaledInput=0  ExternalReset=none  TrackingMode=off  Kt=1  LimitOutput=off  UpperSaturationLimit=inf  LowerSaturationLimit=-inf  LinearizeAsGain=on  AntiWindupMode=none  Kb=1  POutMin=[]  POutMax=[]  IOutMin=[]  IOutMax=[]  DOutMin=[]  DOutMax=[]  NOutMin=[]  NOutMax=[]  SumOutMin=[]  SumOutMax=[]  SaturationOutMin=[]  SaturationOutMax=[]  PParamMin=[]  PParamMax=[]  IParamMin=[]  IParamMax=[]  DParamMin=[]  DParamMax=[]  NParamMin=[]  NParamMax=[]  KbParamMin=[]  KbParamMax=[]  KtParamMin=[]  KtParamMax=[]  KbOutMin=[]  KbOutMax=[]  KtOutMin=[]  KtOutMax=[]  IntegratorOutMin=[]  IntegratorOutMax=[]  FilterOutMin=[]  FilterOutMax=[]  SumI1OutMin=[]  SumI1OutMax=[]  SumI2OutMin=[]  SumI2OutMax=[]  SumI3OutMin=[]  SumI3OutMax=[]  SumI4OutMin=[]  SumI4OutMax=[]  SumDOutMin=[]  SumDOutMax=[]  DifferentiatorOutMin=[]  DifferentiatorOutMax=[]  FilterDiffOutCoefMin=[]  FilterDiffOutCoefMax=[]  ReciprocalOutMin=[]  ReciprocalOutMax=[]  SumDenOutMin=[]  SumDenOutMax=[]  SumNumOutMin=[]  SumNumOutMax=[]  DivideOutMin=[]  DivideOutMax=[]  IntegratorContinuousStateAttributes=''  IntegratorStateMustResolveToSignalObject=off  IntegratorRTWStateStorageClass=Auto  FilterContinuousStateAttributes=''  FilterStateMustResolveToSignalObject=off  FilterRTWStateStorageClass=Auto  ParallelPVariant=InternalParameters  IdealPVariant=Disabled  IVariant=InternalParameters  DVariant=Disabled  IntegratorVariant=Discrete  SatVariant=Disabled  AWVariant=Passthrough  PCopyVariant=Disabled  TRVariant=Disabled  FdbkBlocksVariant=Forward  IdealPFdbkVariant=Disabled  SatFdbkVariant=Disabled  DerivativeFilterVariant=Disabled  NVariant=Disabled  NCopyVariant=Disabled_SignalSpec  FilterICVariant=Disabled  IntegratorICVariant=InternalICs  ExternalResetVariant=Disabled  TRSumVariant=Passthrough  SumFdbkVariant=Disabled  SumVariant=Sum_PI
  PID Control Steering : simulink/Continuous/PID Controller  Controller=PI  Form=Parallel  TimeDomain=Discrete-time  SampleTime=Ts  IntegratorMethod=Forward Euler  FilterMethod=Forward Euler  ControllerParametersSource=internal  P=P_steer  I=I_steer  D=0  UseFilter=on  N=100  TunerSelectOption=Transfer Function Based (PID Tuner App)  InitialConditionSource=internal  InitialConditionForIntegrator=0  InitialConditionForFilter=0  DifferentiatorICPrevScaledInput=0  ExternalReset=none  TrackingMode=off  Kt=1  LimitOutput=off  UpperSaturationLimit=inf  LowerSaturationLimit=-inf  LinearizeAsGain=on  AntiWindupMode=none  Kb=1  POutMin=[]  POutMax=[]  IOutMin=[]  IOutMax=[]  DOutMin=[]  DOutMax=[]  NOutMin=[]  NOutMax=[]  SumOutMin=[]  SumOutMax=[]  SaturationOutMin=[]  SaturationOutMax=[]  PParamMin=[]  PParamMax=[]  IParamMin=[]  IParamMax=[]  DParamMin=[]  DParamMax=[]  NParamMin=[]  NParamMax=[]  KbParamMin=[]  KbParamMax=[]  KtParamMin=[]  KtParamMax=[]  KbOutMin=[]  KbOutMax=[]  KtOutMin=[]  KtOutMax=[]  IntegratorOutMin=[]  IntegratorOutMax=[]  FilterOutMin=[]  FilterOutMax=[]  SumI1OutMin=[]  SumI1OutMax=[]  SumI2OutMin=[]  SumI2OutMax=[]  SumI3OutMin=[]  SumI3OutMax=[]  SumI4OutMin=[]  SumI4OutMax=[]  SumDOutMin=[]  SumDOutMax=[]  DifferentiatorOutMin=[]  DifferentiatorOutMax=[]  FilterDiffOutCoefMin=[]  FilterDiffOutCoefMax=[]  ReciprocalOutMin=[]  ReciprocalOutMax=[]  SumDenOutMin=[]  SumDenOutMax=[]  SumNumOutMin=[]  SumNumOutMax=[]  DivideOutMin=[]  DivideOutMax=[]  IntegratorContinuousStateAttributes=''  IntegratorStateMustResolveToSignalObject=off  IntegratorRTWStateStorageClass=Auto  FilterContinuousStateAttributes=''  FilterStateMustResolveToSignalObject=off  FilterRTWStateStorageClass=Auto  ParallelPVariant=InternalParameters  IdealPVariant=Disabled  IVariant=InternalParameters  DVariant=Disabled  IntegratorVariant=Discrete  SatVariant=Disabled  AWVariant=Passthrough  PCopyVariant=Disabled  TRVariant=Disabled  FdbkBlocksVariant=Forward  IdealPFdbkVariant=Disabled  SatFdbkVariant=Disabled  DerivativeFilterVariant=Disabled  NVariant=Disabled  NCopyVariant=Disabled_SignalSpec  FilterICVariant=Disabled  IntegratorICVariant=InternalICs  ExternalResetVariant=Disabled  TRSumVariant=Passthrough  SumFdbkVariant=Disabled  SumVariant=Sum_PI
  Sum1 : Sum  Inputs=|++
  Sum2 : Sum  Inputs=|++
  Sum4 : Sum  Inputs=+--
  Sum5 : Sum  Inputs=|+-
  Reference Steering Angle : Outport
  wires:
  Lateral Error/1(Lateral Error) -> PID Control Lateral Position/1  "Lateral Error"
  Sum5/1 -> PID Control Steering/1  "Delta Error"
  Estimated Position/1 -> " "/2
  " "/1 -> Lateral Error/2(Position Error (X,Y))  "Position Error"
  Sum4/1 -> PID Control Direction/1  "Delta Reference = Psi Sigma - Nu"
  Measured Steering Angle/1 -> Gain/1
  Estimated Heading/1 -> Sum4/3
  Gain/1 -> Sum5/2
  Gain1/1 -> Gain3/1, Sum4/2
  PID Control Lateral Position/1 -> Gain1/1
  Sum1/1 -> Gain5/1, Sum5/1
  PID Control Steering/1 -> Gain4/1  "Delta Reference"
  Sum2/1 -> Reference Steering Angle/1
  Gain4/1 -> Sum2/1
  Reference Heading/1 -> Lateral Error/1(Psi Sigma), Sum4/1
  Reference Position/1 -> " "/1
  PID Control Direction/1 -> Gain2/1
  Gain2/1 -> Sum1/1
  Gain3/1 -> Sum1/2
  Gain5/1 -> Sum2/2

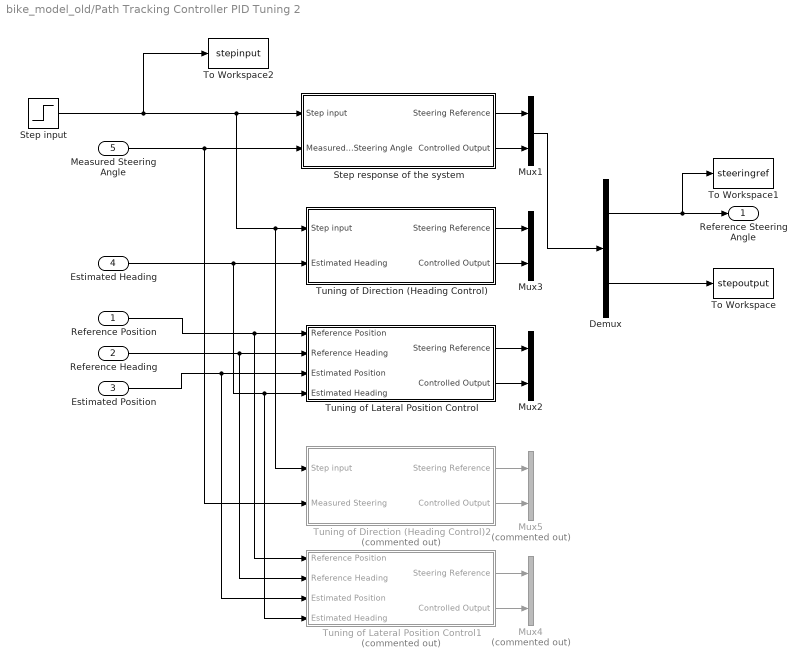
== system bike_model_old/Path Tracking Controller PID Tuning 2 ==
  Reference Position : Inport
  Reference Heading : Inport  Port=2
  Estimated Position : Inport  Port=3
  Estimated Heading : Inport  Port=4
  Measured Steering Angle : Inport  Port=5
  Demux : Demux  Outputs=2
  Mux1 : Mux  Inputs=2
  Mux2 : Mux  Inputs=2
  Mux3 : Mux  Inputs=2
  Mux4 : Mux  Commented=on  Inputs=2
  Mux5 : Mux  Commented=on  Inputs=2
  Step input : Step  Time=15  After=deg2rad(2)  SampleTime=0
  Step response of the system : Subsystem
  To Workspace : ToWorkspace  VariableName=stepoutput  SaveFormat=Timeseries  SampleTime=-1
  To Workspace1 : ToWorkspace  VariableName=steeringref  SaveFormat=Timeseries  SampleTime=-1
  To Workspace2 : ToWorkspace  VariableName=stepinput  SaveFormat=Timeseries  SampleTime=-1
  Tuning of Direction (Heading Control) : Subsystem
  Tuning of Direction (Heading Control)2 : Subsystem  Commented=on
  Tuning of Lateral Position Control : Subsystem
  Tuning of Lateral Position Control1 : Subsystem  Commented=on
  Reference Steering Angle : Outport
  wires:
  Measured Steering Angle/1 -> Tuning of Direction (Heading Control)2/2(Measured Steering), Step response of the system/2(Measured Steering Angle)
  Estimated Heading/1 -> Tuning of Lateral Position Control1/4(Estimated Heading), Tuning of Lateral Position Control/4(Estimated Heading), Tuning of Direction (Heading Control)/2(Estimated Heading)
  Demux/2 -> To Workspace/1
  Demux/1 -> To Workspace1/1, Reference Steering Angle/1
  Step response of the system/1(Steering Reference) -> Mux1/1
  Step response of the system/2(Controlled Output) -> Mux1/2
  Tuning of Lateral Position Control/1(Steering Reference) -> Mux2/1
  Tuning of Direction (Heading Control)/2(Controlled Output) -> Mux3/2
  Tuning of Direction (Heading Control)/1(Steering Reference) -> Mux3/1
  Tuning of Lateral Position Control/2(Controlled Output) -> Mux2/2
  Mux1/1 -> Demux/1
  Reference Heading/1 -> Tuning of Lateral Position Control1/2(Reference Heading), Tuning of Lateral Position Control/2(Reference Heading)
  Estimated Position/1 -> Tuning of Lateral Position Control1/3(Estimated Position), Tuning of Lateral Position Control/3(Estimated Position)
  Reference Position/1 -> Tuning of Lateral Position Control1/1(Reference Position), Tuning of Lateral Position Control/1(Reference Position)
  Step input/1 -> Tuning of Direction (Heading Control)2/1(Step input), Tuning of Direction (Heading Control)/1(Step input), Step response of the system/1(Step input), To Workspace2/1
  Tuning of Direction (Heading Control)2/2(Controlled Output) -> Mux5/2
  Tuning of Direction (Heading Control)2/1(Steering Reference) -> Mux5/1
  Tuning of Lateral Position Control1/2(Controlled Output) -> Mux4/2
  Tuning of Lateral Position Control1/1(Steering Reference) -> Mux4/1

== system bike_model_old/Path Tracking Controller1 ==
  note: Direction Control
  note: Lateral Control
  note: Steering Control
  note: Switch Direct Control
  note: Switch Lateral Control
  Reference Position : Inport
  Reference Heading : Inport  Port=2
  Estimated Position : Inport  Port=3
  Estimated Heading : Inport  Port=4
  " " : Sum  Inputs=|-+
  Gain1 : Gain  Gain=lat_control
  Gain2 : Gain  Gain=direct_control
  Gain3 : Gain  Gain=1-direct_control
  Lateral Error : Subsystem  SystemSampleTime=Ts
  PID Control Lateral Position : simulink/Continuous/PID Controller  Controller=PI  Form=Parallel  TimeDomain=Discrete-time  SampleTime=Ts  IntegratorMethod=Forward Euler  FilterMethod=Forward Euler  ControllerParametersSource=internal  P=P_lat  I=I_lat  D=0  UseFilter=on  N=100  TunerSelectOption=Transfer Function Based (PID Tuner App)  InitialConditionSource=internal  InitialConditionForIntegrator=0  InitialConditionForFilter=0  DifferentiatorICPrevScaledInput=0  ExternalReset=none  TrackingMode=off  Kt=1  LimitOutput=off  UpperSaturationLimit=inf  LowerSaturationLimit=-inf  LinearizeAsGain=on  AntiWindupMode=none  Kb=1  POutMin=[]  POutMax=[]  IOutMin=[]  IOutMax=[]  DOutMin=[]  DOutMax=[]  NOutMin=[]  NOutMax=[]  SumOutMin=[]  SumOutMax=[]  SaturationOutMin=[]  SaturationOutMax=[]  PParamMin=[]  PParamMax=[]  IParamMin=[]  IParamMax=[]  DParamMin=[]  DParamMax=[]  NParamMin=[]  NParamMax=[]  KbParamMin=[]  KbParamMax=[]  KtParamMin=[]  KtParamMax=[]  KbOutMin=[]  KbOutMax=[]  KtOutMin=[]  KtOutMax=[]  IntegratorOutMin=[]  IntegratorOutMax=[]  FilterOutMin=[]  FilterOutMax=[]  SumI1OutMin=[]  SumI1OutMax=[]  SumI2OutMin=[]  SumI2OutMax=[]  SumI3OutMin=[]  SumI3OutMax=[]  SumI4OutMin=[]  SumI4OutMax=[]  SumDOutMin=[]  SumDOutMax=[]  DifferentiatorOutMin=[]  DifferentiatorOutMax=[]  FilterDiffOutCoefMin=[]  FilterDiffOutCoefMax=[]  ReciprocalOutMin=[]  ReciprocalOutMax=[]  SumDenOutMin=[]  SumDenOutMax=[]  SumNumOutMin=[]  SumNumOutMax=[]  DivideOutMin=[]  DivideOutMax=[]  IntegratorContinuousStateAttributes=''  IntegratorStateMustResolveToSignalObject=off  IntegratorRTWStateStorageClass=Auto  FilterContinuousStateAttributes=''  FilterStateMustResolveToSignalObject=off  FilterRTWStateStorageClass=Auto  ParallelPVariant=InternalParameters  IdealPVariant=Disabled  IVariant=InternalParameters  DVariant=Disabled  IntegratorVariant=Discrete  SatVariant=Disabled  AWVariant=Passthrough  PCopyVariant=Disabled  TRVariant=Disabled  FdbkBlocksVariant=Forward  IdealPFdbkVariant=Disabled  SatFdbkVariant=Disabled  DerivativeFilterVariant=Disabled  NVariant=Disabled  NCopyVariant=Disabled_SignalSpec  FilterICVariant=Disabled  IntegratorICVariant=InternalICs  ExternalResetVariant=Disabled  TRSumVariant=Passthrough  SumFdbkVariant=Disabled  SumVariant=Sum_PI
  PID Control Direction : simulink/Continuous/PID Controller  Controller=PI  Form=Parallel  TimeDomain=Discrete-time  SampleTime=Ts  IntegratorMethod=Forward Euler  FilterMethod=Forward Euler  ControllerParametersSource=internal  P=P_direct  I=I_direct  D=0  UseFilter=on  N=100  TunerSelectOption=Transfer Function Based (PID Tuner App)  InitialConditionSource=internal  InitialConditionForIntegrator=0  InitialConditionForFilter=0  DifferentiatorICPrevScaledInput=0  ExternalReset=none  TrackingMode=off  Kt=1  LimitOutput=off  UpperSaturationLimit=inf  LowerSaturationLimit=-inf  LinearizeAsGain=on  AntiWindupMode=none  Kb=1  POutMin=[]  POutMax=[]  IOutMin=[]  IOutMax=[]  DOutMin=[]  DOutMax=[]  NOutMin=[]  NOutMax=[]  SumOutMin=[]  SumOutMax=[]  SaturationOutMin=[]  SaturationOutMax=[]  PParamMin=[]  PParamMax=[]  IParamMin=[]  IParamMax=[]  DParamMin=[]  DParamMax=[]  NParamMin=[]  NParamMax=[]  KbParamMin=[]  KbParamMax=[]  KtParamMin=[]  KtParamMax=[]  KbOutMin=[]  KbOutMax=[]  KtOutMin=[]  KtOutMax=[]  IntegratorOutMin=[]  IntegratorOutMax=[]  FilterOutMin=[]  FilterOutMax=[]  SumI1OutMin=[]  SumI1OutMax=[]  SumI2OutMin=[]  SumI2OutMax=[]  SumI3OutMin=[]  SumI3OutMax=[]  SumI4OutMin=[]  SumI4OutMax=[]  SumDOutMin=[]  SumDOutMax=[]  DifferentiatorOutMin=[]  DifferentiatorOutMax=[]  FilterDiffOutCoefMin=[]  FilterDiffOutCoefMax=[]  ReciprocalOutMin=[]  ReciprocalOutMax=[]  SumDenOutMin=[]  SumDenOutMax=[]  SumNumOutMin=[]  SumNumOutMax=[]  DivideOutMin=[]  DivideOutMax=[]  IntegratorContinuousStateAttributes=''  IntegratorStateMustResolveToSignalObject=off  IntegratorRTWStateStorageClass=Auto  FilterContinuousStateAttributes=''  FilterStateMustResolveToSignalObject=off  FilterRTWStateStorageClass=Auto  ParallelPVariant=InternalParameters  IdealPVariant=Disabled  IVariant=InternalParameters  DVariant=Disabled  IntegratorVariant=Discrete  SatVariant=Disabled  AWVariant=Passthrough  PCopyVariant=Disabled  TRVariant=Disabled  FdbkBlocksVariant=Forward  IdealPFdbkVariant=Disabled  SatFdbkVariant=Disabled  DerivativeFilterVariant=Disabled  NVariant=Disabled  NCopyVariant=Disabled_SignalSpec  FilterICVariant=Disabled  IntegratorICVariant=InternalICs  ExternalResetVariant=Disabled  TRSumVariant=Passthrough  SumFdbkVariant=Disabled  SumVariant=Sum_PI
  Sum1 : Sum  Inputs=|++
  Sum4 : Sum  Inputs=+--
  Reference Steering Angle : Outport
  wires:
  Lateral Error/1(Lateral Error) -> PID Control Lateral Position/1  "Lateral Error"
  Estimated Position/1 -> " "/2
  " "/1 -> Lateral Error/2(Position Error (X,Y))  "Position Error"
  Sum4/1 -> PID Control Direction/1  "Delta Reference = Psi Sigma - Nu"
  Estimated Heading/1 -> Sum4/3
  Gain1/1 -> Gain3/1, Sum4/2
  PID Control Lateral Position/1 -> Gain1/1
  Reference Heading/1 -> Lateral Error/1(Psi Sigma), Sum4/1
  Reference Position/1 -> " "/1
  PID Control Direction/1 -> Gain2/1
  Gain2/1 -> Sum1/1
  Gain3/1 -> Sum1/2
  Sum1/1 -> Reference Steering Angle/1

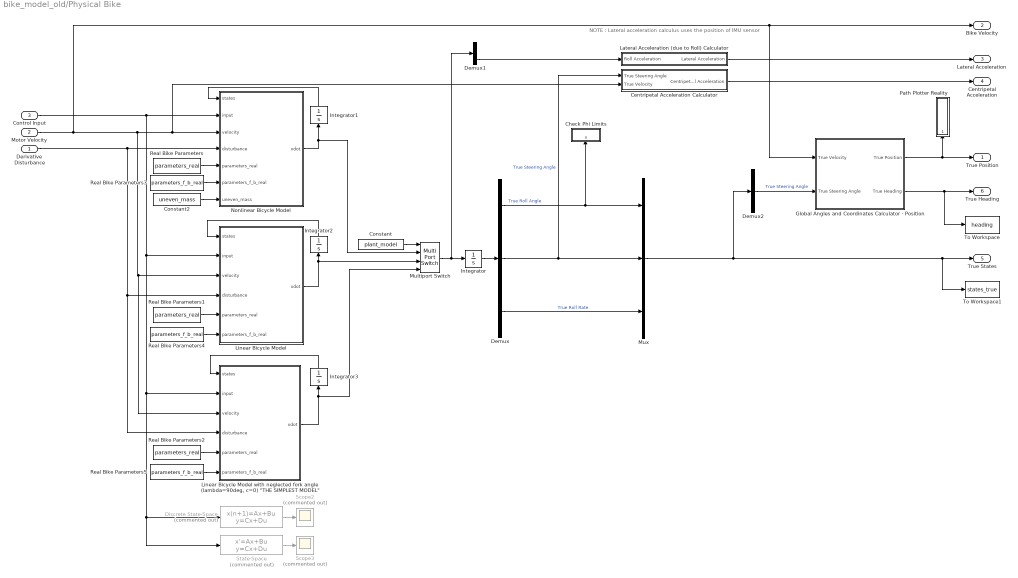
== system bike_model_old/Physical Bike ==
  note: NOTE : Lateral acceleration calculus uses the position of IMU sensor
  Derivative Disturbance : Inport
  Motor Velocity : Inport  Port=2
  Control Input : Inport  Port=3
  Centripetal Acceleration Calculator : Subsystem
  Check Phi Limits : Subsystem  TreatAsAtomicUnit=on  SystemSampleTime=Ts
  Constant : Constant  Value=plant_model
  Constant2 : Constant  Value=uneven_mass
  Demux : Demux  Outputs=3
  Demux1 : Demux  Outputs=3
  Demux2 : Demux  Outputs=3
  Discrete State-Space : DiscreteStateSpace  Commented=on  A=sys_dis.A  B=sys_dis.B  C=eye(3,3)  D=zeros(3,1)  SampleTime=Ts_IMU
  Global Angles and Coordinates Calculator - Position : Subsystem  SystemSampleTime=Ts
  Integrator{,1..3} (4 alike) : Integrator  InitialCondition=initial_states
  Lateral Acceleration (due to Roll) Calculator : Subsystem
  Linear Bicycle Model : MATLAB Function  TreatAsAtomicUnit=on
  "Linear Bicycle Model with neglected fork angle (lambda=90deg, c=0) \"THE SIMPLEST MODEL\"" : MATLAB Function  TreatAsAtomicUnit=on
  Multiport Switch : MultiPortSwitch
  Mux : Mux  Inputs=3
  Nonlinear Bicycle Model : MATLAB Function  TreatAsAtomicUnit=on
  Path Plotter Reality : Subsystem  SystemSampleTime=Ts
  Real Bike Parameters : Constant  Value=parameters_real
  Real Bike Parameters1 : Constant  Value=parameters_real
  Real Bike Parameters2 : Constant  Value=parameters_real
  Real Bike Parameters3 : Constant  Value=parameters_f_b_real
  Real Bike Parameters4 : Constant  Value=parameters_f_b_real
  Real Bike Parameters5 : Constant  Value=parameters_f_b_real
  Scope2 : Scope  Commented=on
  Scope3 : Scope  Commented=on
  State-Space : StateSpace  Commented=on  A=sys_con.A  B=sys_con.B  C=eye(3,3)  D=zeros(3,1)  InitialCondition=0
  To Workspace : ToWorkspace  VariableName=heading  SaveFormat=Timeseries  SampleTime=Ts
  To Workspace1 : ToWorkspace  VariableName=states_true  SaveFormat=Timeseries  SampleTime=Ts
  True Position : Outport
  Bike Velocity : Outport  Port=2
  Lateral Acceleration : Outport  Port=3
  Centripetal Acceleration : Outport  Port=4
  True States : Outport  Port=5
  True Heading : Outport  Port=6
  wires:
  Real Bike Parameters5/1 -> "Linear Bicycle Model with neglected fork angle (lambda=90deg, c=0) \"THE SIMPLEST MODEL\""/6(parameters_f_b_real)
  Demux/2 -> Mux/2, Centripetal Acceleration Calculator/1(True Steering Angle)  "True Steering Angle"
  Control Input/1 -> State-Space/1, Discrete State-Space/1, "Linear Bicycle Model with neglected fork angle (lambda=90deg, c=0) \"THE SIMPLEST MODEL\""/2(input), Linear Bicycle Model/2(input), Nonlinear Bicycle Model/2(input)
  Integrator1/1 -> Nonlinear Bicycle Model/1(states)
  Real Bike Parameters3/1 -> Nonlinear Bicycle Model/6(parameters_f_b_real)
  Constant/1 -> Multiport Switch/1
  Real Bike Parameters2/1 -> "Linear Bicycle Model with neglected fork angle (lambda=90deg, c=0) \"THE SIMPLEST MODEL\""/5(parameters_real)
  State-Space/1 -> Scope3/1
  Discrete State-Space/1 -> Scope2/1
  Integrator/1 -> Demux/1
  Demux/1 -> Mux/1, Check Phi Limits/1(x)  "True Roll Angle"
  Real Bike Parameters1/1 -> Linear Bicycle Model/5(parameters_real)
  Centripetal Acceleration Calculator/1(Centripetal Acceleration) -> Centripetal Acceleration/1
  Nonlinear Bicycle Model/1(xdot) -> Integrator1/1, Multiport Switch/2
  Demux1/3 -> Lateral Acceleration (due to Roll) Calculator/1(Roll Acceleration)
  Linear Bicycle Model/1(xdot) -> Integrator2/1, Multiport Switch/3
  Derivative Disturbance/1 -> "Linear Bicycle Model with neglected fork angle (lambda=90deg, c=0) \"THE SIMPLEST MODEL\""/4(disturbance), Linear Bicycle Model/4(disturbance), Nonlinear Bicycle Model/4(disturbance)
  Real Bike Parameters/1 -> Nonlinear Bicycle Model/5(parameters_real)
  "Linear Bicycle Model with neglected fork angle (lambda=90deg, c=0) \"THE SIMPLEST MODEL\""/1(xdot) -> Integrator3/1, Multiport Switch/4
  Multiport Switch/1 -> Demux1/1, Integrator/1
  Lateral Acceleration (due to Roll) Calculator/1(Lateral Acceleration) -> Lateral Acceleration/1
  Integrator3/1 -> "Linear Bicycle Model with neglected fork angle (lambda=90deg, c=0) \"THE SIMPLEST MODEL\""/1(states)
  Integrator2/1 -> Linear Bicycle Model/1(states)
  Motor Velocity/1 -> "Linear Bicycle Model with neglected fork angle (lambda=90deg, c=0) \"THE SIMPLEST MODEL\""/3(velocity), Linear Bicycle Model/3(velocity), Nonlinear Bicycle Model/3(velocity), Centripetal Acceleration Calculator/2(True Velocity), Global Angles and Coordinates Calculator - Position/1(True Velocity), Bike Velocity/1
  Real Bike Parameters4/1 -> Linear Bicycle Model/6(parameters_f_b_real)
  Demux/3 -> Mux/3  "True Roll Rate"
  Mux/1 -> To Workspace1/1, True States/1, Demux2/1
  Demux2/2 -> Global Angles and Coordinates Calculator - Position/2(True Steering Angle)  "True Steering Angle"
  Global Angles and Coordinates Calculator - Position/1(True Position) -> True Position/1, Path Plotter Reality/1(Position)
  Global Angles and Coordinates Calculator - Position/2(True Heading) -> True Heading/1, To Workspace/1
  Constant2/1 -> Nonlinear Bicycle Model/7(uneven_mass)

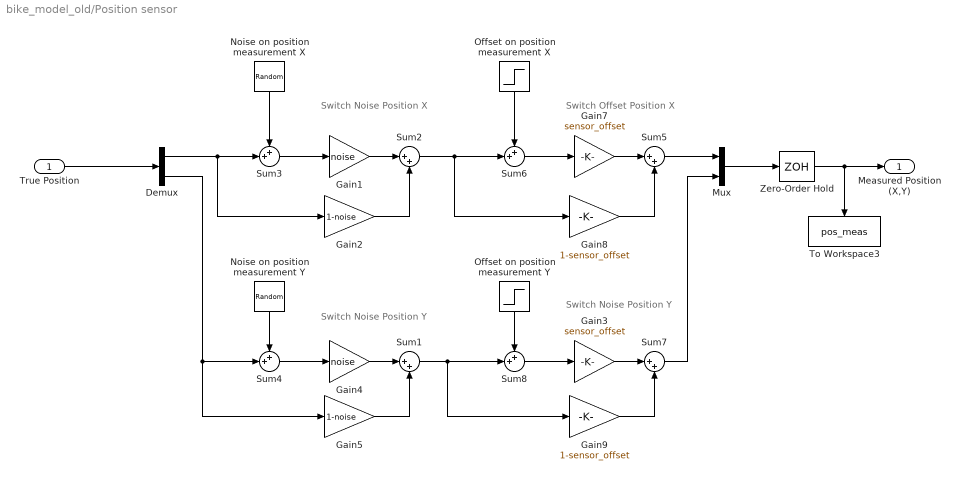
== system bike_model_old/Position sensor ==
  note: Switch Noise
      | Position X
  note: Switch Noise
      | Position Y
  note: Switch Offset
      | Position X
  note: Switch Noise
      | Position Y
  True Position : Inport
  Demux : Demux  Outputs=2
  Gain1 : Gain  Gain=noise
  Gain2 : Gain  Gain=1-noise
  Gain3 : Gain  Gain=sensor_offset
  Gain4 : Gain  Gain=noise
  Gain5 : Gain  Gain=1-noise
  Gain7 : Gain  Gain=sensor_offset
  Gain8 : Gain  Gain=1-sensor_offset
  Gain9 : Gain  Gain=1-sensor_offset
  Mux : Mux  Inputs=2
  "Noise on position measurement X    " : RandomNumber  Variance=noise_pos_meas  Seed=2  SampleTime=Ts
  "Noise on position measurement Y     " : RandomNumber  Variance=noise_pos_meas  SampleTime=Ts
  "Offset on position measurement X    " : Step  Time=time_offset_pos_x  After=offset_pos_x  SampleTime=Ts
  "Offset on position measurement Y     " : Step  Time=time_offset_pos_y  After=offset_pos_y  SampleTime=Ts
  Sum{1..2,5,7} (4 alike) : Sum  Inputs=|++
  Sum{3..4,6,8} (4 alike) : Sum  Inputs=++|
  To Workspace3 : ToWorkspace  VariableName=pos_meas  SaveFormat=Timeseries  SampleTime=-1
  Zero-Order Hold : ZeroOrderHold  SampleTime=Ts
  "Measured Position (X,Y) " : Outport
  wires:
  Zero-Order Hold/1 -> To Workspace3/1, "Measured Position (X,Y) "/1
  True Position/1 -> Demux/1
  Mux/1 -> Zero-Order Hold/1
  "Noise on position measurement X    "/1 -> Sum3/1
  Demux/1 -> Gain2/1, Sum3/2
  "Noise on position measurement Y     "/1 -> Sum4/1
  Demux/2 -> Sum4/2, Gain5/1
  Sum3/1 -> Gain1/1
  Gain1/1 -> Sum2/1
  Gain4/1 -> Sum1/1
  Sum4/1 -> Gain4/1
  Gain2/1 -> Sum2/2
  Gain5/1 -> Sum1/2
  Sum2/1 -> Sum6/2, Gain8/1
  "Offset on position measurement X    "/1 -> Sum6/1
  Sum6/1 -> Gain7/1
  Gain8/1 -> Sum5/2
  Gain7/1 -> Sum5/1
  Sum5/1 -> Mux/1
  Gain3/1 -> Sum7/1
  Sum8/1 -> Gain3/1
  "Offset on position measurement Y     "/1 -> Sum8/1
  Sum1/1 -> Gain9/1, Sum8/2
  Gain9/1 -> Sum7/2
  Sum7/1 -> Mux/2
